simulink model "ep4_6_1"  (R2018a)
settings: Solver=VariableStepAuto  StartTime=0.0  StopTime=20  MaxStep=0.001  RelTol=1e-3
settings Model: Creator=zheny  LastModifiedBy=zheny

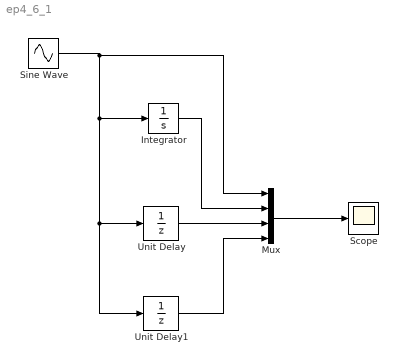
== system ep4_6_1 ==
  Integrator : Integrator
  Mux : Mux
  Scope : Scope
  Sine Wave : Sin  SampleTime=0
  Unit Delay : UnitDelay  SampleTime=0.5
  Unit Delay1 : UnitDelay  SampleTime=1.2
  wires:
  Mux/1 -> Scope/1
  Sine Wave/1 -> Mux/1, Unit Delay1/1, Unit Delay/1, Integrator/1
  Integrator/1 -> Mux/2
  Unit Delay/1 -> Mux/3
  Unit Delay1/1 -> Mux/4
